simulink model "BEML_EMU"  (R2019b)
settings: configuration reference "ConfigSet_SimIntegration" (kept outside this file)
model workspace (MAT data in the model file):
  BrakesSampleTime = 0.01
  ConfigSampleTime = 0.05
  CouplingSampleTime = 0.05
  DoorsSampleTime = 0.05
  DynamicsSampleTime = 0.001
  ElectricalSampleTime = 0.05
  PRM_SimIntegration : Simulink.Parameter (value not decoded)
  PantographSampleTime = 0.05
  PneumaticsSampleTime = 0.01
  SampleTime = 0.001
  TractionSampleTime = 0.01
undefined symbols (not defined in the file): Acceleration, AngularAcceleration, AngularVelocity, BrakeFadeEnable, Brakes, BrakeShoeCoefficientCalculationMethod, BrakeShoeFrictionCoeff, BrakeTemperatureEnable, Common, DampingAdjustmentDesignMass, DavisCoeffA1, DavisCoeffA2, DavisCoeffB1, DavisCoeffB2, DavisCoefficients, DavisCoeffLeadCarC, DavisCoeffTailCarC, DiscIntNeverNeededParam, Doors, DragCalculationMethod, Dynamics, Effects, Electrical, EnableDampingAdjustmentByMass, Environment, Equipment, ExternalEffects, H, HasMotor, HasPanto, HornActivation, IsFirstVehicle, IsLastVehicle, isLeft, IsNonCab, LateralJolt, Location, LongitudinalJolt, MaxVehicles, MotionBaseSafetyCutout, OrientationDCM, P, Pantograph, Pneumatics, PneumaticsPoweredPanto, R, Traction, Transform, Tuning, UnitConfig, Velocity, VerticalJolt, VerticalJoltDown, VigilanceIntervention
libraries: simulink x35, IOStateMachinesLib x26, TestBenchLib x6, LatchesLib x3, BEML_EMU_BrakesInput_Lib x1, BEML_EMU_CBTCInterface_Lib x1, BEML_EMU_Couplers_Lib x1, BEML_EMU_DoorsInput_Lib x1, BEML_EMU_DynamicsInput_Lib x1, BEML_EMU_ElectricalInput_Lib x1, BEML_EMU_PantographInput_Lib x1, BEML_EMU_PneumaticsInput_Lib x1
(part 6 of 6)

== system BEML_EMU/InputsInterface/VehicleConfigProcessing/VehicleConfigInterface/VehicleConfigInterface/LocationConfig/UnitConf ==
  In Bus Element1 : Inport  PortName=VehicleConfig  Element=Class
  In Bus Element2 : Inport  PortName=VehicleConfig  Element=Enabled
  ClassDown : Inport  Port=2
  ClassUp : Inport  Port=3
  Compare To Constant : simulink/Logic and Bit Operations/Compare To Constant  relop===  const=102  OutDataTypeStr=boolean
  Compare To Constant1 : simulink/Logic and Bit Operations/Compare To Constant  relop===  const=101  OutDataTypeStr=boolean
  Compare To Constant{2,4,8..9} (4 alike) : simulink/Logic and Bit Operations/Compare To Constant  relop===  const=103  OutDataTypeStr=boolean
  Compare To Constant5 : simulink/Logic and Bit Operations/Compare To Constant  relop===  const=102  OutDataTypeStr=boolean
  Data Type Conversion : DataTypeConversion
  Data Type Conversion1 : DataTypeConversion
  Logical Operator : Logic  AllPortsSameDT=off  OutDataTypeStr=boolean
  Logical Operator2 : Logic  Inputs=3  AllPortsSameDT=off  OutDataTypeStr=boolean
  Logical Operator4 : Logic  AllPortsSameDT=off  OutDataTypeStr=boolean
  Logical Operator5 : Logic  Operator=OR  Inputs=3  AllPortsSameDT=off  OutDataTypeStr=boolean
  Logical Operator6 : Logic  AllPortsSameDT=off  OutDataTypeStr=boolean
  Logical Operator7 : Logic  Operator=NOT  AllPortsSameDT=off  OutDataTypeStr=boolean
  UnitConnection : Outport  VectorParamsAs1DForOutWhenUnconnected=off
  Enabled : Outport  Port=2  VectorParamsAs1DForOutWhenUnconnected=off
  wires:
  In Bus Element1/1 -> Data Type Conversion/1
  Data Type Conversion/1 -> Compare To Constant9/1, Compare To Constant5/1, Compare To Constant1/1  "VehicleClasEnum"
  Logical Operator5/1 -> Logical Operator7/1
  ClassDown/1 -> Compare To Constant4/1, Compare To Constant/1
  Compare To Constant/1 -> Logical Operator/1
  Compare To Constant1/1 -> Logical Operator/2
  Compare To Constant4/1 -> Logical Operator2/1
  Compare To Constant5/1 -> Logical Operator2/2
  Compare To Constant8/1 -> Logical Operator4/1
  Compare To Constant9/1 -> Logical Operator4/2
  Logical Operator/1 -> Logical Operator5/1
  Logical Operator2/1 -> Logical Operator5/2
  Logical Operator4/1 -> Logical Operator5/3
  Logical Operator7/1 -> Logical Operator6/2
  In Bus Element2/1 -> Logical Operator6/1, Data Type Conversion1/1
  Data Type Conversion1/1 -> Enabled/1
  Logical Operator6/1 -> UnitConnection/1
  Compare To Constant2/1 -> Logical Operator2/3
  ClassUp/1 -> Compare To Constant8/1, Compare To Constant2/1

== system BEML_EMU/SimulatorSystems/ScoringSystemInterface/TrainLevelScoring/For Each Subsystem/Subsystem/Subsystem ==
  <Bogie> : Inport  Partition=on  PartitionDimension=1  PartitionWidth=1  PartitionOffset=0
  Bus Selector2 : BusSelector  OutputSignals=TractionPower,EDBrakingPower
  Discrete-Time Integrator : DiscreteIntegrator  SampleTime=-1  ICPrevOutput=DiscIntNeverNeededParam  ICPrevScaledInput=DiscIntNeverNeededParam
  Discrete-Time Integrator1 : DiscreteIntegrator  SampleTime=-1  ICPrevOutput=DiscIntNeverNeededParam  ICPrevScaledInput=DiscIntNeverNeededParam
  For Each : ForEach  DisableCoverage=on
  Out1 : Outport  ConcatenationDimension=1
  Out2 : Outport  Port=2  ConcatenationDimension=1
  wires:
  Bus Selector2/1 -> Discrete-Time Integrator/1  "<TractionPower>"
  Discrete-Time Integrator/1 -> Out1/1
  <Bogie>/1 -> Bus Selector2/1
  Bus Selector2/2 -> Discrete-Time Integrator1/1  "<EDBrakingPower>"
  Discrete-Time Integrator1/1 -> Out2/1

== system BEML_EMU/SimulatorSystems/Subsystem/Input Adapter/MotionBaseInputAdapter/Vehicle Dynamics In Processing/Coordinate Transformations ==
  Heave : Inport
  Pitch : Inport  Port=2
  Bus Assignment2 : BusAssignment  AssignedSignals=OrientationDCM,H,P,R
  Constant8 : Constant  Value=0  OutDataTypeStr=Bus: BD_MotionBase_In_Vehicle_Dynamics_Transform
  Orientation DCM : Subsystem
  Roll : Constant  Value=0
  Transform : Outport
  wires:
  Heave/1 -> Orientation DCM/1(Heave), Bus Assignment2/3  "H"
  Bus Assignment2/1 -> Transform/1
  Pitch/1 -> Orientation DCM/2(Pitch), Bus Assignment2/4  "P"
  Roll/1 -> Bus Assignment2/5  "R"
  Constant8/1 -> Bus Assignment2/1
  Orientation DCM/1(DCM) -> Bus Assignment2/2  "OrientationDCM"

== system BEML_EMU/InputsInterface/VehicleConfigProcessing/VehicleConfigInterface/VehicleConfigInterface/AssignElectrical/VehicleEquipment/If Action Subsystem ==
  In1 : Inport
  Action Port : ActionPort  ActionPortLabel=if(u1<=1)
  Bus Assignment3 : BusAssignment  AssignedSignals=IsDM1
  Constant : Constant  OutDataTypeStr=Inherit: Inherit via back propagation
  Out1 : Outport
  wires:
  Bus Assignment3/1 -> Out1/1
  In1/1 -> Bus Assignment3/1
  Constant/1 -> Bus Assignment3/2

== system BEML_EMU/InputsInterface/VehicleConfigProcessing/VehicleConfigInterface/VehicleConfigInterface/AssignElectrical/VehicleEquipment/If Action Subsystem1 ==
  In1 : Inport
  Action Port : ActionPort  ActionPortLabel=else
  Bus Assignment3 : BusAssignment  AssignedSignals=IsDM3
  Constant : Constant  OutDataTypeStr=Inherit: Inherit via back propagation
  Out1 : Outport
  wires:
  Constant/1 -> Bus Assignment3/2
  In1/1 -> Bus Assignment3/1
  Bus Assignment3/1 -> Out1/1

== system BEML_EMU/InputsInterface/VehicleConfigProcessing/VehicleConfigInterface/VehicleConfigInterface/AssignElectrical/VehicleEquipment/If Action Subsystem2 ==
  In1 : Inport
  Action Port : ActionPort  ActionPortLabel=elseif(u1<=5)
  Bus Assignment3 : BusAssignment  AssignedSignals=IsDM2
  Constant : Constant  OutDataTypeStr=Inherit: Inherit via back propagation
  Out1 : Outport
  wires:
  Bus Assignment3/1 -> Out1/1
  In1/1 -> Bus Assignment3/1
  Constant/1 -> Bus Assignment3/2

== system BEML_EMU/InputsInterface/VehicleConfigProcessing/VehicleConfigInterface/VehicleConfigInterface/AssignElectrical/VehicleEquipment1/If Action Subsystem ==
  In1 : Inport
  Action Port : ActionPort  ActionPortLabel=if(u1<=2)
  Bus Assignment3 : BusAssignment  AssignedSignals=IsT1
  Constant : Constant  OutDataTypeStr=Inherit: Inherit via back propagation
  Out1 : Outport
  wires:
  Bus Assignment3/1 -> Out1/1
  In1/1 -> Bus Assignment3/1
  Constant/1 -> Bus Assignment3/2

== system BEML_EMU/InputsInterface/VehicleConfigProcessing/VehicleConfigInterface/VehicleConfigInterface/AssignElectrical/VehicleEquipment1/If Action Subsystem1 ==
  In1 : Inport
  Action Port : ActionPort  ActionPortLabel=elseif(u1<=4)
  Bus Assignment3 : BusAssignment  AssignedSignals=IsT2
  Constant : Constant  OutDataTypeStr=Inherit: Inherit via back propagation
  Out1 : Outport
  wires:
  Constant/1 -> Bus Assignment3/2
  In1/1 -> Bus Assignment3/1
  Bus Assignment3/1 -> Out1/1

== system BEML_EMU/InputsInterface/VehicleConfigProcessing/VehicleConfigInterface/VehicleConfigInterface/AssignElectrical/VehicleEquipment1/If Action Subsystem2 ==
  In1 : Inport
  Action Port : ActionPort  ActionPortLabel=else
  Bus Assignment3 : BusAssignment  AssignedSignals=IsT3
  Constant : Constant  OutDataTypeStr=Inherit: Inherit via back propagation
  Out1 : Outport
  wires:
  Bus Assignment3/1 -> Out1/1
  In1/1 -> Bus Assignment3/1
  Constant/1 -> Bus Assignment3/2

== system BEML_EMU/InputsInterface/VehicleConfigProcessing/VehicleConfigInterface/VehicleConfigInterface/AssignElectrical/VehicleEquipment3/If Action Subsystem ==
  In1 : Inport
  Action Port : ActionPort  ActionPortLabel=if(u1<=2)
  Bus Assignment3 : BusAssignment  AssignedSignals=IsM1
  Constant : Constant  OutDataTypeStr=Inherit: Inherit via back propagation
  Out1 : Outport
  wires:
  Bus Assignment3/1 -> Out1/1
  In1/1 -> Bus Assignment3/1
  Constant/1 -> Bus Assignment3/2

== system BEML_EMU/InputsInterface/VehicleConfigProcessing/VehicleConfigInterface/VehicleConfigInterface/AssignElectrical/VehicleEquipment3/If Action Subsystem1 ==
  In1 : Inport
  Action Port : ActionPort  ActionPortLabel=elseif(u1<=4)
  Bus Assignment3 : BusAssignment  AssignedSignals=IsM2
  Constant : Constant  OutDataTypeStr=Inherit: Inherit via back propagation
  Out1 : Outport
  wires:
  Constant/1 -> Bus Assignment3/2
  In1/1 -> Bus Assignment3/1
  Bus Assignment3/1 -> Out1/1

== system BEML_EMU/InputsInterface/VehicleConfigProcessing/VehicleConfigInterface/VehicleConfigInterface/AssignElectrical/VehicleEquipment3/If Action Subsystem2 ==
  In1 : Inport
  Action Port : ActionPort  ActionPortLabel=else
  Bus Assignment3 : BusAssignment  AssignedSignals=IsM3
  Constant : Constant  OutDataTypeStr=Inherit: Inherit via back propagation
  Out1 : Outport
  wires:
  Bus Assignment3/1 -> Out1/1
  In1/1 -> Bus Assignment3/1
  Constant/1 -> Bus Assignment3/2

== system BEML_EMU/SimulatorSystems/Subsystem/Input Adapter/MotionBaseInputAdapter/Vehicle Dynamics In Processing/Coordinate Transformations/Orientation DCM ==
  Heave : Inport
  Pitch : Inport  Port=2
  Heave Matrix : Subsystem
  Matrix Multiply : Product  Multiplication=Matrix(*)
  Pitch Matrix : Subsystem
  DCM : Outport
  wires:
  Pitch/1 -> Pitch Matrix/1(Pitch)
  Pitch Matrix/1(Heave Transform) -> Matrix Multiply/1
  Heave/1 -> Heave Matrix/1(Heave)
  Heave Matrix/1(Heave Transform) -> Matrix Multiply/2
  Matrix Multiply/1 -> DCM/1

== system BEML_EMU/SimulatorSystems/Subsystem/Input Adapter/MotionBaseInputAdapter/Vehicle Dynamics In Processing/Coordinate Transformations/Orientation DCM/Heave Matrix ==
  Heave : Inport
  Add : Sum  Inputs=+++
  Constant : Constant  Value=[0 0 0; 0 0 0; 0 0 1]
  Gain : Gain  Gain=[0 -1 0; 1 0 0; 0 0 0]
  Gain2 : Gain  Gain=[1 0 0; 0 1 0; 0 0 0]
  Trigonometric Function : Trigonometry
  Trigonometric Function1 : Trigonometry  Operator=cos
  Heave Transform : Outport
  wires:
  Gain2/1 -> Add/2
  Heave/1 -> Trigonometric Function1/1, Trigonometric Function/1
  Constant/1 -> Add/3
  Add/1 -> Heave Transform/1  "Heave Transform"
  Gain/1 -> Add/1
  Trigonometric Function/1 -> Gain/1
  Trigonometric Function1/1 -> Gain2/1

== system BEML_EMU/SimulatorSystems/Subsystem/Input Adapter/MotionBaseInputAdapter/Vehicle Dynamics In Processing/Coordinate Transformations/Orientation DCM/Pitch Matrix ==
  Pitch : Inport
  Add1 : Sum  Inputs=+++
  Constant1 : Constant  Value=[0 0 0; 0 1 0; 0 0 0]
  Gain1 : Gain  Gain=[1 0 0; 0 0 0; 0 0 1]
  Gain3 : Gain  Gain=[0 0 1; 0 0 0; -1 0 0]
  Trigonometric Function2 : Trigonometry
  Trigonometric Function3 : Trigonometry  Operator=cos
  Heave Transform : Outport
  wires:
  Pitch/1 -> Trigonometric Function3/1, Trigonometric Function2/1
  Gain1/1 -> Add1/2
  Trigonometric Function3/1 -> Gain1/1
  Constant1/1 -> Add1/3
  Add1/1 -> Heave Transform/1  "Heave Transform"
  Trigonometric Function2/1 -> Gain3/1
  Gain3/1 -> Add1/1
